simulink model "verify_DHW_Energy_Tapping_mdl"  (R2016b)
settings: Solver=ode45  StartTime=0.0  StopTime=24*3600  MaxStep=100  RelTol=1e-3  EnableMultiTasking=on
libraries: carnot x6
settings Model: Creator=drhf  LastModifiedBy=srrt
settings DataIOCC: SaveFormat=Array  SignalLoggingSaveFormat=ModelDataLogs
settings OptimizationCC: ExpressionDepthLimit=2147483647  LifeSpan=inf
settings DebuggingCC: UnderspecifiedInitializationDetection=Classic  MergeDetectMultiDrivingBlocksExec=none  SolverPrmCheckMsg=warning  FcnCallInpInsideContextMsg=warning  StateNameClashWarn=warning  SFUnexpectedBacktrackingDiag=warning  SFNoUnconditionalDefaultTransitionDiag=warning  SFExecutionAtInitializationDiag=none
settings HardwareCC: ProdBitPerPointer=32  ProdBitPerSizeT=32  ProdBitPerPtrDiffT=32  ProdLargestAtomicFloat=None  ProdIntDivRoundTo=Undefined  ProdEndianess=Unspecified  ProdWordSize=32  ProdHWDeviceType=32-bit Generic
settings ModelReferenceCC: PropagateSignalLabelsOutOfModel=off
settings GRTTargetCC: TargetLangStandard=C89/C90 (ANSI)  GeneratePreprocessorConditionals=Disable all  CombineOutputUpdateFcns=off  GRTInterface=on
settings ConfigComp: CovMetricSettings=dw  CovHtmlReporting=on  CovSaveCumulativeToWorkspaceVar=on  CovSaveSingleToWorkspaceVar=on  CovExternalEMLEnable=off

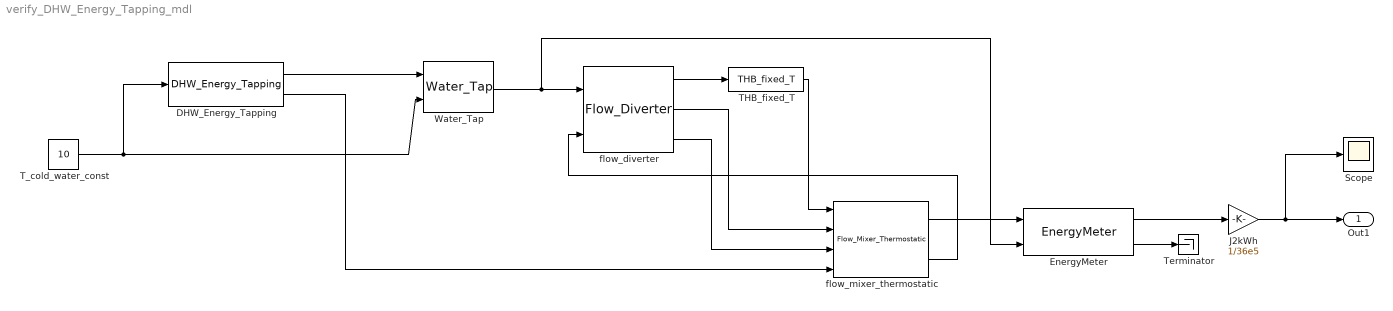
== system verify_DHW_Energy_Tapping_mdl ==
  DHW_Energy_Tapping : carnot/Load/Hot_Water_Tapping/DHW_Energy_Tapping  mdot_nom=1/60  times="[7     7.1 7.5   8.083 8.25  8.5   8.75  9     9.5   10.5  11.5  11.75 12.75 14.5  15.5  16.5  18    18.25 18.5  19    20.5  21.25 21.5]*3600"  energies=[0.105 1.4 0.105 0.105 0.105 0.105 0.105 0.105 0.105 0.105 0.105 0.105 0.315 0.105 0.105 0.105 0.105 0.105 0.105 0.105 0.735 0.105 1.4 ]*36e5  dT_set="[30    30  30    30    30    30    30    30    30    30    30    30    45    30    30    30    30    30    30    30    45    30    30  ]"  coeffs="[3     6   3     3     3     3     3     3     3     3     3     3     4     3     3     3     3     3     3     3     4     3     6   ]"
  EnergyMeter : carnot/Control/EnergyMeter
  J2kWh : Gain  Gain=1/36e5
  Scope : Scope
  THB_fixed_T : carnot/Source/Simple/THB_fixed_T  t=60
  T_cold_water_const : Constant  Value=10
  Terminator : Terminator
  Water_Tap : carnot/Load/Hot_Water_Tapping/Water_Tap  dia=0.02  p=2e5
  flow_diverter : carnot/Hydraulics/Flow_Diverter
  flow_mixer_thermostatic : carnot/Hydraulics/Flow_Mixer_Thermostatic  t=10
  Out1 : Outport
  wires:
  T_cold_water_const/1 -> Water_Tap/2, DHW_Energy_Tapping/1
  flow_diverter/3 -> flow_mixer_thermostatic/3
  flow_diverter/2 -> flow_mixer_thermostatic/2
  THB_fixed_T/1 -> flow_mixer_thermostatic/1
  flow_mixer_thermostatic/2 -> flow_diverter/2
  Water_Tap/1 -> EnergyMeter/2, flow_diverter/1
  flow_diverter/1 -> THB_fixed_T/1
  DHW_Energy_Tapping/1 -> Water_Tap/1
  DHW_Energy_Tapping/2 -> flow_mixer_thermostatic/4
  flow_mixer_thermostatic/1 -> EnergyMeter/1
  EnergyMeter/1 -> J2kWh/1
  J2kWh/1 -> Scope/1, Out1/1
  EnergyMeter/2 -> Terminator/1
